simulink model "MotorXploer_NOW_"  (R2025a)
settings: Solver=FixedStepAuto  StartTime=0.0  StopTime=inf  FixedStep=0.001  RelTol=1e-3
undefined symbols (not defined in the file): Blocking, LF, Non
libraries: amg_usbconverter_n_connect_lib x3, dspstat3 x2, dspfdesign x1, simulink x1
settings Model: Creator=beamk  LastModifiedBy=Palm

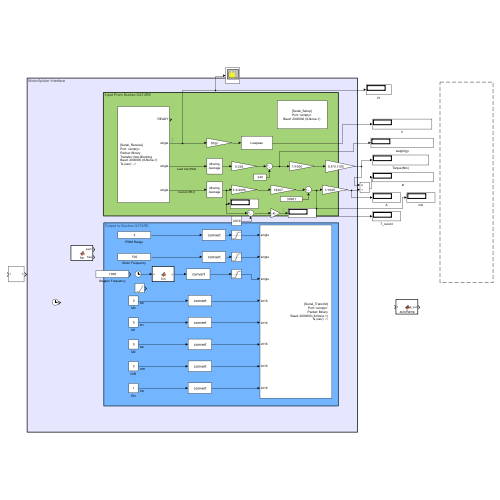
[thumbnail: Simulink's stored preview of the top-level diagram]
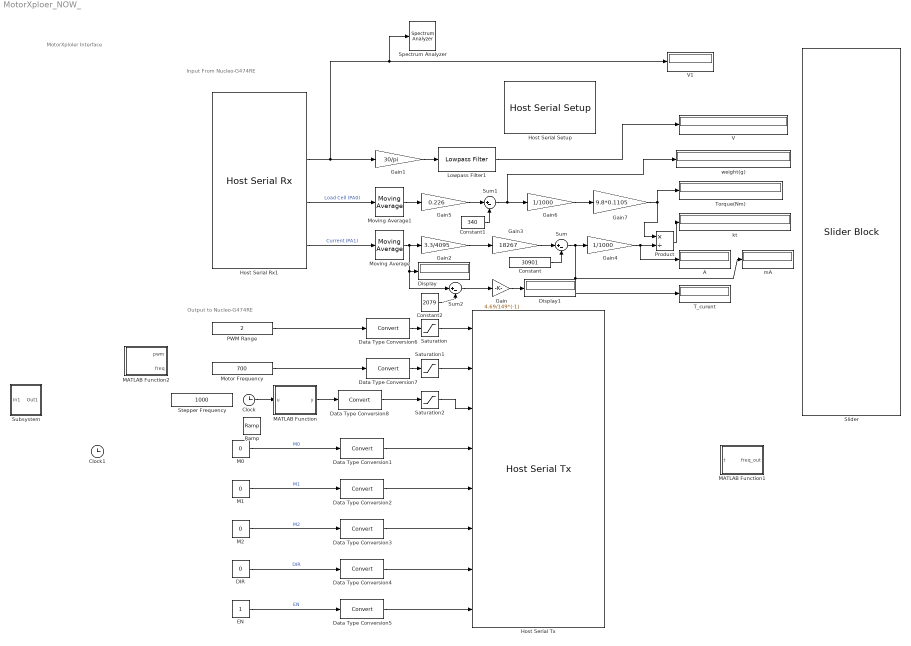
== system MotorXploer_NOW_ ==
  note: Output to Nucleo-G474RE
  note: Input From Nucleo-G474RE
  note: MotorXploler Interface
  A : Display
  Clock : Clock
  Clock1 : Clock
  Constant : Constant  Value=30901
  Constant1 : Constant  Value=340
  Constant2 : Constant  Value=2079
  DIR : Constant  Value=0
  Data Type Conversion{1..8} (8 alike) : DataTypeConversion  SaturateOnIntegerOverflow=off  RndMeth=Floor
  Display : Display
  Display1 : Display
  EN : Constant
  Gain : Gain  Gain=4.69/149*(-1)
  Gain1 : Gain  Gain=30/pi
  Gain2 : Gain  Gain=3.3/4095
  Gain3 : Gain  Gain=18267
  Gain4 : Gain  Gain=1/1000
  Gain5 : Gain  Gain=0.226
  Gain6 : Gain  Gain=1/1000
  Gain7 : Gain  Gain=9.8*0.1105
  Host Serial Rx1 : amg_usbconverter_n_connect_lib/Host Serial Rx  conf=rx  port=<auto>  baudrate=2000000  databits=8  parity=None  stopbit=1  flowcontrol=None  transfer=Non-Blocking  timeout=5  packetmode=Binary  enableinitialvalues=off  initialvalues=[]  binheader='25'  binterminator='4E'  porttype_double=0  porttype_single=3  porttype_int8=0  porttype_uint8=0  porttype_int16=0  porttype_uint16=0  porttype_int32=0  porttype_uint32=0  asciiformat='%f,%f,%d,%d'  rx_asciiterminator="LF (0x0A - \"\\n\")"  tx_asciiterminator="CRLF (0x0D 0x0A - \"\\r\\n\")"  sampletime=-1  enablecustomportlabel=off  cinputportlabel=0  coutputportlabel=A  portpinstr=0  blockid=HostSerialRx1  inputporttype=[]  inputportwidth=[]  inputportlabel={}  outputporttype=[3 1 1 1]  outputportwidth=[1 1 1 1]  outputportlabel={'READY','single','single','single'}  compat=0  optionstring=[]  autoport='<empty>'
  Host Serial Setup : amg_usbconverter_n_connect_lib/Host Serial Setup  conf=setup  port=<auto>  baudrate=2000000  databits=8  parity=None  stopbit=1  flowcontrol=None  transfer=Blocking  timeout=2  packetmode=Binary  initialvalues=[]  binheader='7E 7E'  binterminator='03 03'  porttype_double=0  porttype_single=1  porttype_int8=0  porttype_uint8=0  porttype_int16=0  porttype_uint16=0  porttype_int32=0  porttype_uint32=2  asciiformat='%d %u %x'  rx_asciiterminator="CRLF (0x0D 0x0A - \"\\r\\n\")"  tx_asciiterminator="CRLF (0x0D 0x0A - \"\\r\\n\")"  sampletime=-1  enablecustomportlabel=off  cinputportlabel=0  coutputportlabel=A  portpinstr=0  blockid=HostSerialSetup  inputporttype=[]  inputportwidth=[]  inputportlabel={}  outputporttype=[]  outputportwidth=[]  outputportlabel={}  compat=0  optionstring=[]  autoport='<empty>'
  Host Serial Tx : amg_usbconverter_n_connect_lib/Host Serial Tx  conf=tx  port=<auto>  baudrate=2000000  databits=8  parity=None  stopbit=1  flowcontrol=None  transfer=Blocking  timeout=2  packetmode=Binary  initialvalues=[]  binheader='25'  binterminator='4E'  porttype_double=0  porttype_single=3  porttype_int8=0  porttype_uint8=0  porttype_int16=5  porttype_uint16=0  porttype_int32=0  porttype_uint32=0  asciiformat='%d,%f'  rx_asciiterminator="CRLF (0x0D 0x0A - \"\\r\\n\")"  tx_asciiterminator="CRLF (0x0D 0x0A - \"\\r\\n\")"  sampletime=-1  enablecustomportlabel=off  cinputportlabel=0  coutputportlabel=A  portpinstr=0  blockid=HostSerialTx  inputporttype=[1 1 1 4 4 4 4 4]  inputportwidth=[1 1 1 1 1 1 1 1]  inputportlabel={'single','single','single','int16','int16','int16','int16','int16'}  outputporttype=[]  outputportwidth=[]  outputportlabel={}  compat=0  optionstring=[]  autoport='<empty>'
      settings: SourceProductName=aMG USB Converter N
  Lowpass Filter1 : dspfdesign/Lowpass Filter  FilterType=FIR  DesignForMinimumOrder=on  FilterOrder=50  PassbandFrequency=0.03  StopbandFrequency=0.1  PassbandRipple=0.1  StopbandAttenuation=80  SampleRateMode=Use normalized frequency (0 to 1)  SampleRate=44100  SimulateUsing=Interpreted execution  roundingMode=Floor  coeffsDataTypeStr=fixdt(1,16)
  M0 : Constant  Value=0
  M1 : Constant  Value=0
  M2 : Constant  Value=0
  MATLAB Function : MATLAB Function  TreatAsAtomicUnit=on
  MATLAB Function1 : MATLAB Function  TreatAsAtomicUnit=on
  MATLAB Function2 : MATLAB Function  TreatAsAtomicUnit=on
  Motor Frequency : Constant  Value=700  OutDataTypeStr=single
  Moving Average : dspstat3/Moving Average  Method=Sliding window  ForgettingFactorPort=off  SpecifyWindowLength=on  WindowLength=4  OverlapLength=3  AllowArbitraryInputLength=off  ForgettingFactor=0.9  SimulateUsing=Interpreted execution
  Moving Average1 : dspstat3/Moving Average  Method=Sliding window  ForgettingFactorPort=off  SpecifyWindowLength=on  WindowLength=4  OverlapLength=3  AllowArbitraryInputLength=off  ForgettingFactor=0.9  SimulateUsing=Interpreted execution
  PWM Range : Constant  Value=2  OutDataTypeStr=single
  Product : Product  Inputs=*/
  Ramp : simulink/Sources/Ramp  slope=100  start=0  InitialOutput=0
  Saturation : Saturate  UpperLimit=65535  LowerLimit=-65535
  Saturation1 : Saturate  UpperLimit=20000  LowerLimit=0
  Saturation2 : Saturate  UpperLimit=inf  LowerLimit=0
  Slider : SliderBlock  ScaleMin=-100
  Spectrum Analyzer : SpectrumAnalyzer  WindowPosition=[441.000000,33.000000,800.000000,500.000000,]  ScopeFrameLocation=window  SampleRate=44.1e3  PlotAsTwoSidedSpectrum=off  FrequencyScale=Log  WindowInvariantSamplesPerUpdate=on  FrequencySpan=Start and stop frequencies  StartFrequency=0  StopFrequency=500  YLimits=[-3603.4449 -2802.6794]  SelectedToolstripTab=spectrumAnalyzerToolstrip.estimationTab
  Stepper Frequency : Constant  Value=1000  OutDataTypeStr=single
  Subsystem : Subsystem
  Sum : Sum  Inputs=|+-
  Sum1 : Sum  Inputs=|+-
  Sum2 : Sum  Inputs=|+-
  T_curent : Display
  Torque(Nm) : Display
  V : Display
  V1 : Display
  kt : Display
  mA : Display
  weight(g) : Display
  wires:
  Host Serial Rx1/2 -> Gain1/1, Spectrum Analyzer/1, V1/1
  Host Serial Rx1/3 -> Moving Average1/1  "Load Cell (PA0)"
  M0/1 -> Data Type Conversion1/1  "M0"
  EN/1 -> Data Type Conversion5/1  "EN"
  DIR/1 -> Data Type Conversion4/1  "DIR"
  M1/1 -> Data Type Conversion2/1  "M1"
  M2/1 -> Data Type Conversion3/1  "M2"
  Data Type Conversion1/1 -> Host Serial Tx/4
  Data Type Conversion2/1 -> Host Serial Tx/5
  Data Type Conversion3/1 -> Host Serial Tx/6
  Data Type Conversion4/1 -> Host Serial Tx/7
  Data Type Conversion5/1 -> Host Serial Tx/8
  Data Type Conversion6/1 -> Saturation/1
  Saturation/1 -> Host Serial Tx/1
  Data Type Conversion7/1 -> Saturation1/1
  Data Type Conversion8/1 -> Saturation2/1
  Saturation1/1 -> Host Serial Tx/2
  Saturation2/1 -> Host Serial Tx/3
  Host Serial Rx1/4 -> Moving Average/1  "Current (PA1)"
  Moving Average/1 -> Sum2/1, Display/1, Gain2/1
  Gain2/1 -> Gain3/1
  Gain3/1 -> Sum/1
  Constant/1 -> Sum/2
  Sum/1 -> T_curent/1, mA/1, Gain4/1
  Gain1/1 -> Lowpass Filter1/1
  Lowpass Filter1/1 -> V/1
  Moving Average1/1 -> Gain5/1
  Gain5/1 -> Sum1/1
  Constant1/1 -> Sum1/2
  Sum1/1 -> weight(g)/1, Gain6/1
  Gain6/1 -> Gain7/1
  Gain7/1 -> Product/1, Torque(Nm)/1
  Gain4/1 -> A/1, Product/2
  Product/1 -> kt/1
  Clock/1 -> MATLAB Function/1(u)
  MATLAB Function/1(y) -> Data Type Conversion8/1
  Constant2/1 -> Sum2/2
  Sum2/1 -> Gain/1
  Gain/1 -> Display1/1
  PWM Range/1 -> Data Type Conversion6/1
  Motor Frequency/1 -> Data Type Conversion7/1

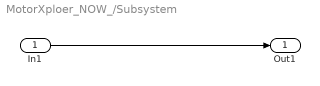
== system MotorXploer_NOW_/Subsystem ==
  In1 : Inport
  Out1 : Outport
  wires:
  In1/1 -> Out1/1

== matlab function MotorXploer_NOW_/MATLAB Function ==
  data: u input; y output
function y = fcn(u)

% u = time (from Simulink clock)

% output y = frequency (0 → 15000 Hz, step 1500 Hz, repeat)

persistent freq_index

% initialize on first run

if isempty(freq_index)

freq_index = 0;

end

% Each step lasts 1 second (10 steps = 10 seconds)

step_duration = 0.5; % second

% Step number (0 → 9)

step_number = floor(u / step_duration);

% Wrap around every 10 steps

freq_index = mod(step_number, 25);

% Output frequency

y = freq_index * 60; % 0,1500,...,15000

== matlab function MotorXploer_NOW_/MATLAB Function2 ==
  data: pwm output; freq output
function [pwm, freq] = fcn()

persistent freqList pwmStep sampleCount freqIndex pwmIndex roundCount;

% Initialize
if isempty(freqList)
    freqList = [5000 10000 15000 20000];
    pwmStep = 0:0.2:1.0; 
    %pwmStep = 0:0.1:1.0; 
    sampleCount = 0;
    freqIndex = 1;
    pwmIndex = 1;
    roundCount = 1;
end

% Stop after 4 rounds
if roundCount > 1
    pwm = 0;
    freq = 0;
    return;
end

% Output 
freq = freqList(freqIndex);
pwm  = pwmStep(pwmIndex) * (-65535);   % <-- ตอนนี้เป็น double แล้ว

% Update counter
sampleCount = sampleCount + 1;

if sampleCount >= 10000
    sampleCount = 0;
    pwmIndex = pwmIndex + 1;

    if pwmIndex > length(pwmStep)
        pwmIndex = 1;
        freqIndex = freqIndex + 1;

        if freqIndex > length(freqList)
            freqIndex = 1;
            roundCount = roundCount + 1;
        end
    end
end

== matlab function MotorXploer_NOW_/MATLAB Function1 ==
  data: t input; freq_out output
function freq_out = autoRamp(t)
% auto increase frequency with correct timing
persistent freq_now last_t

startDelay = 1.0;      % รอ 1 วินาทีแล้วค่อยเริ่ม
rampRate   = 100;      % เพิ่ม 100 Hz ต่อ 1 วินาที
maxFreq    = 10000;     % จำกัด max (ปรับได้)

% Init
if isempty(freq_now)
    freq_now = 0;
    last_t = t;
end

% ก่อนถึงเวลาเริ่ม → ส่ง 0
if t < startDelay
    freq_now = 0;
    last_t = t;
    freq_out = 0;
    return;
end

% คำนวณ dt จริงจาก Simulink (ไม่ต้องเดา)
dt = t - last_t;
last_t = t;

% ป้องกัน dt เพี้ยน/โดด
if dt < 0 || dt > 0.1
    dt = 0;
end

% Ramp (ขึ้นลื่นตามเวลาจริง)
freq_now = freq_now + rampRate * dt;

% จำกัดไม่ให้เกินความถี่สูงสุด
if freq_now > maxFreq
    freq_now = maxFreq;
end

freq_out = freq_now;
